simulink model "IRB140"  (R2019a)
settings: Solver=VariableStepAuto  StartTime=0.0  StopTime=10.0  RelTol=1e-3
InitFcn:
  | rpm_max=5000;
  | trq_stall=7;
  | T_i=1e-3;
  | eta=100;
  | rpm_eta=3000;
  | trq_eta=2.07;
  | J=0.672*1e-4;
  | rpm0=0;
  | gearRatio=10;
  | ts=0.0025;
undefined symbols (not defined in the file or in its folder): sigbuilder_block, X, Y, Z
libraries: sm_lib x61, fl_lib x42, nesl_utility x31, simulink x12, eeGeneralControl x12, ee_lib x6
(part 1 of 3)
settings Model: Creator=Richard urben  LastModifiedBy=Richard urben

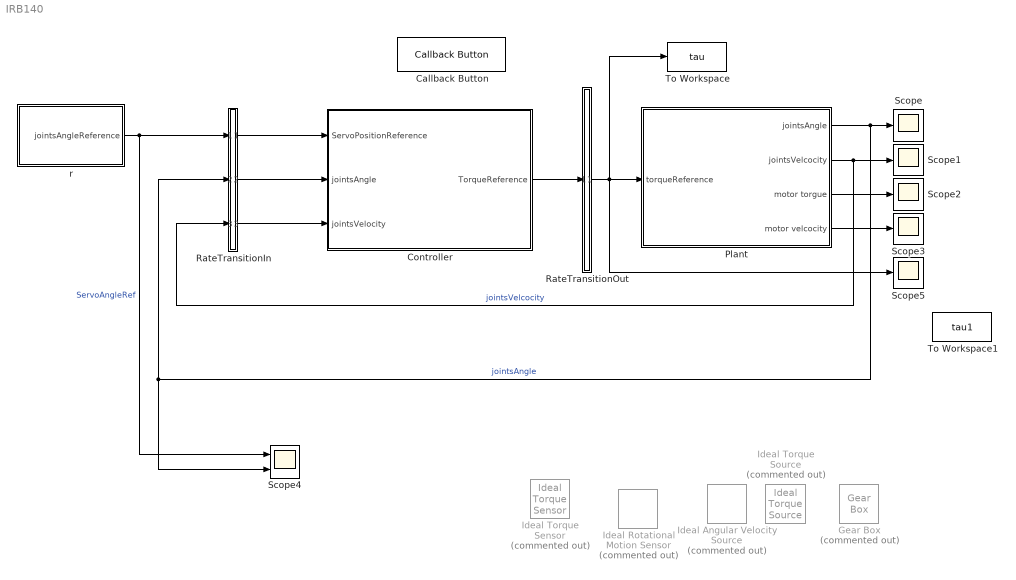
== system IRB140 ==
  Callback Button : CallbackButton  ButtonText=controler tuner
      settings: ClickFcn=|
      | h=0.005;
      | k=0.5;
      | controlParameters;
      | controlSystemTuner('ControlSystemTunerSession.mat');
  Controller : Subsystem
  Gear Box : fl_lib/Mechanical/Mechanisms/Gear Box  Commented=on  ratio=5  t_in_specify=off  t_in_priority=None  t_in=0 N*m  t_in_nominal_specify=off  t_in_nominal_unit=N*m  t_in_nominal_value=1  t_out_specify=off  t_out_priority=None  t_out=0 N*m  t_out_nominal_specify=off  t_out_nominal_unit=N*m  t_out_nominal_value=1
  Ideal Angular Velocity Source : fl_lib/Mechanical/Mechanical Sources/Ideal Angular Velocity Source  Commented=on
  Ideal Rotational Motion Sensor : fl_lib/Mechanical/Mechanical Sensors/Ideal Rotational Motion Sensor  Commented=on  offset=0 rad
  Ideal Torque Sensor : fl_lib/Mechanical/Mechanical Sensors/Ideal Torque Sensor  Commented=on
  Ideal Torque Source : fl_lib/Mechanical/Mechanical Sources/Ideal Torque Source  Commented=on
  Plant : Subsystem
  RateTransitionIn : Subsystem
  RateTransitionOut : Subsystem
  Scope{,1..3,5} (5 alike) : Scope
  Scope4 : Scope  NumInputPorts=2
  To Workspace : ToWorkspace  VariableName=tau  SaveFormat=Timeseries  SampleTime=2.5e-3
      settings: Decimation=6
  To Workspace1 : ToWorkspace  VariableName=tau1  SaveFormat=Timeseries  SampleTime=2.5e-3
      settings: Decimation=6
  r : Subsystem
      mask Display: disp('input')
  wires:
  Plant/2(jointsVelcocity) -> RateTransitionIn/3(joints_VelocityIn), Scope1/1  "jointsVelcocity"
  RateTransitionOut/1(tRef) -> Scope5/1, To Workspace/1, Plant/1(torqueReference)
  Controller/1(TorqueReference) -> RateTransitionOut/1(tRefIn)
  RateTransitionIn/1(ServoPositionRefOut) -> Controller/1(ServoPositionReference)
  RateTransitionIn/2(joints_AngleOut) -> Controller/2(jointsAngle)
  RateTransitionIn/3(joints_VelocityOut) -> Controller/3(jointsVelocity)
  Plant/1(jointsAngle) -> Scope4/2, RateTransitionIn/2(joints_AngleIn), Scope/1  "jointsAngle"
  r/1(jointsAngleReference) -> Scope4/1, RateTransitionIn/1(ServoPositionRefIn)  "ServoAngleRef"
  Plant/3(motor torgue) -> Scope2/1
  Plant/4(motor velcocity) -> Scope3/1

== system IRB140/Controller ==
  ServoPositionReference : Inport  Unit=deg  SampleTime=ts
  jointsAngle : Inport  Port=2  Unit=deg  SampleTime=ts
  jointsVelocity : Inport  Port=3  Unit=deg/s  SampleTime=ts
  Servomotor Position Controller : Subsystem
  Servomotor Speed Controller : Subsystem
  TorqueReference : Outport  Unit=N*m  SampleTime=ts
  wires:
  Servomotor Speed Controller/1(servo_Tref) -> TorqueReference/1  "Tref"
  jointsAngle/1 -> Servomotor Position Controller/2(joint_q)
  jointsVelocity/1 -> Servomotor Speed Controller/2(joint_qd)
  ServoPositionReference/1 -> Servomotor Position Controller/1(servon_qref)
  Servomotor Position Controller/1(servon_qdref) -> Servomotor Speed Controller/1(servon_qdref)  "servoqdref"

== system IRB140/Plant ==
  torqueReference : Inport  Unit=N*m
  DC Voltage Source : fl_lib/Electrical/Electrical Sources/DC Voltage Source  v0=12 V
  ERef Vcc : fl_lib/Electrical/Electrical Elements/Electrical Reference
      settings: SourceProductName=Foundation Library
  MRRef Motor : fl_lib/Mechanical/Rotational Elements/Mechanical Rotational Reference
      settings: SourceProductName=Foundation Library
  robot : Subsystem
  servo system : Subsystem
  jointsAngle : Outport  Unit=deg
  jointsVelcocity : Outport  Port=2  Unit=deg/s
  motor torgue : Outport  Port=3
  motor velcocity : Outport  Port=4
  wires:
  robot/2(w) -> jointsVelcocity/1  "jointsvelocity"
  robot/1(q) -> jointsAngle/1  "jointsangle"
  servo system/1(torque) -> motor torgue/1  "motor torque"
  servo system/2(motVel) -> motor velcocity/1  "motor velocity"
  torqueReference/1 -> servo system/1(tRef)
  connections:
  robot/LConn4 -- servo system/RConn4
  robot/LConn5 -- servo system/RConn5
  robot/LConn3 -- servo system/RConn3
  robot/LConn1 -- servo system/RConn1
  robot/LConn6 -- servo system/RConn6
  servo system/RConn7 -- MRRef Motor/LConn1 -- robot/LConn7
  robot/LConn2 -- servo system/RConn2
  ERef Vcc/LConn1 -- DC Voltage Source/RConn1 -- servo system/LConn2
  DC Voltage Source/LConn1 -- servo system/LConn1

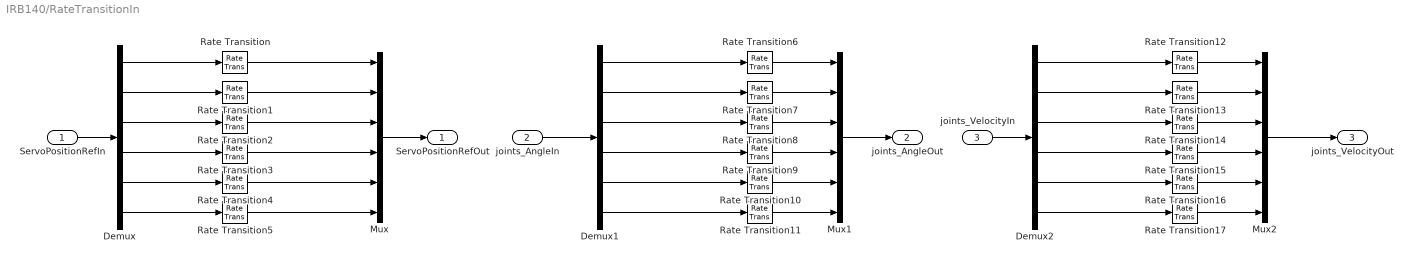
== system IRB140/RateTransitionIn ==
  ServoPositionRefIn : Inport  Unit=deg
  joints_AngleIn : Inport  Port=2  Unit=deg
  joints_VelocityIn : Inport  Port=3
  Demux : Demux  Outputs=6
  Demux1 : Demux  Outputs=6
  Demux2 : Demux  Outputs=6
  Mux : Mux  Inputs=6
  Mux1 : Mux  Inputs=6
  Mux2 : Mux  Inputs=6
  Rate Transition{,1..17} (18 alike) : RateTransition  OutPortSampleTime=ts
  ServoPositionRefOut : Outport
  joints_AngleOut : Outport  Port=2
  joints_VelocityOut : Outport  Port=3
  wires:
  Demux1/6 -> Rate Transition11/1
  Demux1/3 -> Rate Transition8/1
  joints_AngleIn/1 -> Demux1/1
  Demux1/1 -> Rate Transition6/1
  Demux1/5 -> Rate Transition10/1
  Demux/6 -> Rate Transition5/1
  Demux1/4 -> Rate Transition9/1
  Demux/2 -> Rate Transition1/1
  Demux1/2 -> Rate Transition7/1
  Demux/3 -> Rate Transition2/1
  Demux/4 -> Rate Transition3/1
  Demux/1 -> Rate Transition/1
  Demux/5 -> Rate Transition4/1
  Demux2/5 -> Rate Transition16/1
  Demux2/4 -> Rate Transition15/1
  Demux2/3 -> Rate Transition14/1
  Demux2/1 -> Rate Transition12/1
  Demux2/2 -> Rate Transition13/1
  Demux2/6 -> Rate Transition17/1
  Rate Transition/1 -> Mux/1
  Rate Transition1/1 -> Mux/2
  Rate Transition2/1 -> Mux/3
  Rate Transition3/1 -> Mux/4
  Rate Transition4/1 -> Mux/5
  Rate Transition5/1 -> Mux/6
  Mux/1 -> ServoPositionRefOut/1
  Rate Transition7/1 -> Mux1/2
  Rate Transition11/1 -> Mux1/6
  Mux1/1 -> joints_AngleOut/1
  Rate Transition9/1 -> Mux1/4
  Rate Transition6/1 -> Mux1/1
  Rate Transition8/1 -> Mux1/3
  Rate Transition10/1 -> Mux1/5
  Rate Transition12/1 -> Mux2/1
  Rate Transition13/1 -> Mux2/2
  Rate Transition14/1 -> Mux2/3
  Rate Transition15/1 -> Mux2/4
  Rate Transition16/1 -> Mux2/5
  Rate Transition17/1 -> Mux2/6
  Mux2/1 -> joints_VelocityOut/1
  ServoPositionRefIn/1 -> Demux/1
  joints_VelocityIn/1 -> Demux2/1

== system IRB140/RateTransitionOut ==
  tRefIn : Inport  Unit=N*m
  Demux : Demux  Outputs=6
  Mux : Mux  Inputs=6
  Zero-Order Hold{,1..5} (6 alike) : ZeroOrderHold  SampleTime=-1
  tRef : Outport  SampleTime=ts
  wires:
  Demux/3 -> Zero-Order Hold2/1
  tRefIn/1 -> Demux/1
  Demux/2 -> Zero-Order Hold1/1
  Demux/5 -> Zero-Order Hold4/1
  Demux/4 -> Zero-Order Hold3/1
  Demux/1 -> Zero-Order Hold/1
  Demux/6 -> Zero-Order Hold5/1
  Zero-Order Hold5/1 -> Mux/6
  Zero-Order Hold4/1 -> Mux/5
  Zero-Order Hold1/1 -> Mux/2
  Zero-Order Hold/1 -> Mux/1
  Zero-Order Hold2/1 -> Mux/3
  Zero-Order Hold3/1 -> Mux/4
  Mux/1 -> tRef/1

== system IRB140/r ==
  Mux : Mux  Commented=on  Inputs=6
  Mux1 : Mux  Inputs=6
  Subsystem : Subsystem
  Trajectories1 : Subsystem  Tag=STV Subsys  Commented=on  LoadFcn=sigbuilder_block('load');  StartFcn=sigbuilder_block('start');  StopFcn=sigbuilder_block('stop');  ClipboardFcn=sigbuilder_block('clipboard');  mask(Sigbuilder block){tuvar=[0:10]}
      mask help: Simulink:masks:SigbuilderBlock_MD
      mask init:
      | if ~strcmp(get_param(bdroot(gcbh),'SimulationStatus'),'stopped') tuvar = sigbuilder_block('maskInit'); end
      settings: CopyFcn=sigbuilder_block('copy');  DeleteFcn=sigbuilder_block('delete');  ModelCloseFcn=sigbuilder_block('modelClose');  PreSaveFcn=sigbuilder_block('preSave');  PauseFcn=sigbuilder_block('pause');  ContinueFcn=sigbuilder_block('continue');  NameChangeFcn=sigbuilder_block('namechange');  OpenFcn=sigbuilder_block('open',[6 -16.5 1248 598.5 ]);  CloseFcn=sigbuilder_block('close');
      mask Display: plot(0, 0, 100, 100,[2, 2, 32, 32, 2], [68, 8, 8, 68, 68],[32, 2], [38, 38], [32, 19, 2],[53, 60, 44], [32, 17, 17, 2],[16, 16, 31, 31]);txt = getActiveGroup(gcbh);text(2, 100, txt,'verticalAlignment', 'top');
  jointsAngleReference : Outport
  wires:
  Trajectories1/6(servopos6) -> Mux/6
  Trajectories1/2(servopos2) -> Mux/2
  Trajectories1/5(servopos5) -> Mux/5
  Trajectories1/1(servopos1) -> Mux/1
  Trajectories1/4(servopos4) -> Mux/4
  Trajectories1/3(servopos3) -> Mux/3
  Subsystem/5(Out5) -> Mux1/5
  Subsystem/1(Out1) -> Mux1/1
  Subsystem/3(Out3) -> Mux1/3
  Subsystem/2(Out2) -> Mux1/2
  Subsystem/6(Out6) -> Mux1/6
  Subsystem/4(Out4) -> Mux1/4
  Mux1/1 -> jointsAngleReference/1  "jointsAngleReferene"

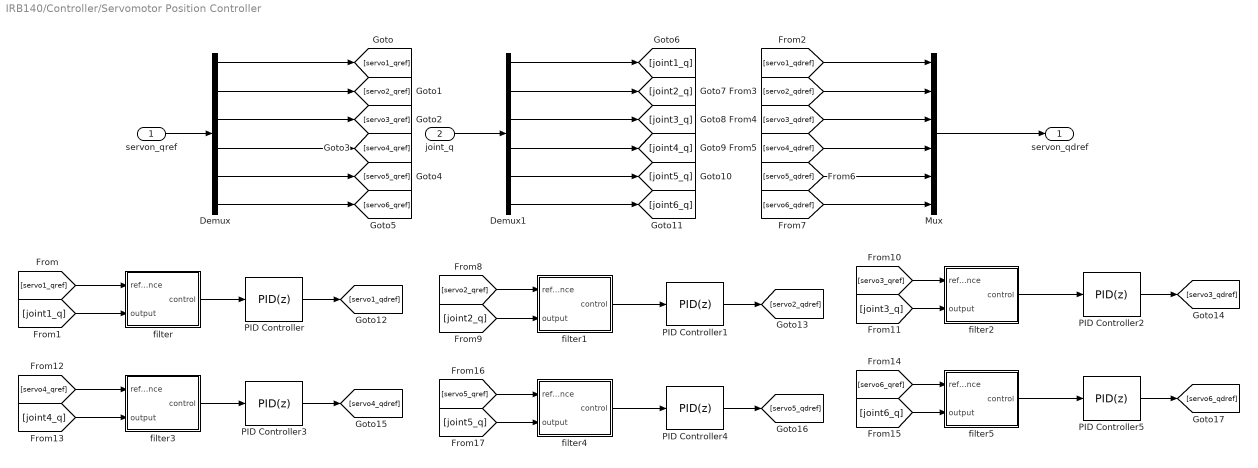
== system IRB140/Controller/Servomotor Position Controller ==
  servon_qref : Inport  Unit=deg
  joint_q : Inport  Port=2  Unit=deg
  Demux : Demux  Outputs=6
  Demux1 : Demux  Outputs=6
  Mux : Mux  Inputs=6
  PID Controller : simulink/Continuous/PID Controller  Controller=PID  Form=Parallel  TimeDomain=Discrete-time  SampleTime=ts  IntegratorMethod=Forward Euler  FilterMethod=Forward Euler  ControllerParametersSource=internal  P=9.61814981930867  I=0.000384969709550726  D=1.05281007023022  UseFilter=on  N=761.904761904762  TunerSelectOption=Transfer Function Based (PID Tuner App)  InitialConditionSource=internal  InitialConditionForIntegrator=0  InitialConditionForFilter=0  DifferentiatorICPrevScaledInput=0  ExternalReset=none  TrackingMode=off  Kt=1  LimitOutput=off  UpperSaturationLimit=inf  LowerSaturationLimit=-inf  LinearizeAsGain=on  AntiWindupMode=none  Kb=1  POutMin=[]  POutMax=[]  IOutMin=[]  IOutMax=[]  DOutMin=[]  DOutMax=[]  NOutMin=[]  NOutMax=[]  SumOutMin=[]  SumOutMax=[]  SaturationOutMin=[]  SaturationOutMax=[]  PParamMin=[]  PParamMax=[]  IParamMin=[]  IParamMax=[]  DParamMin=[]  DParamMax=[]  NParamMin=[]  NParamMax=[]  KbParamMin=[]  KbParamMax=[]  KtParamMin=[]  KtParamMax=[]  KbOutMin=[]  KbOutMax=[]  KtOutMin=[]  KtOutMax=[]  IntegratorOutMin=[]  IntegratorOutMax=[]  FilterOutMin=[]  FilterOutMax=[]  SumI1OutMin=[]  SumI1OutMax=[]  SumI2OutMin=[]  SumI2OutMax=[]  SumI3OutMin=[]  SumI3OutMax=[]  SumI4OutMin=[]  SumI4OutMax=[]  SumDOutMin=[]  SumDOutMax=[]  DifferentiatorOutMin=[]  DifferentiatorOutMax=[]  FilterDiffOutCoefMin=[]  FilterDiffOutCoefMax=[]  ReciprocalOutMin=[]  ReciprocalOutMax=[]  SumDenOutMin=[]  SumDenOutMax=[]  SumNumOutMin=[]  SumNumOutMax=[]  DivideOutMin=[]  DivideOutMax=[]  IntegratorContinuousStateAttributes=''  IntegratorStateMustResolveToSignalObject=off  IntegratorRTWStateStorageClass=Auto  FilterContinuousStateAttributes=''  FilterStateMustResolveToSignalObject=off  FilterRTWStateStorageClass=Auto  ParallelPVariant=InternalParameters  IdealPVariant=Disabled  IVariant=InternalParameters  DVariant=InternalParameters  IntegratorVariant=Discrete  SatVariant=Disabled  AWVariant=Passthrough  PCopyVariant=Disabled  TRVariant=Disabled  FdbkBlocksVariant=Forward  IdealPFdbkVariant=Disabled  SatFdbkVariant=Disabled  DerivativeFilterVariant=ForwardEulerFilter  NVariant=InternalParameters  NCopyVariant=Disabled  FilterICVariant=InternalICsFilter  IntegratorICVariant=InternalICs  ExternalResetVariant=Disabled  TRSumVariant=Passthrough  SumFdbkVariant=Disabled  SumVariant=Sum_PID
  PID Controller1 : simulink/Continuous/PID Controller  Controller=PID  Form=Parallel  TimeDomain=Discrete-time  SampleTime=ts  IntegratorMethod=Forward Euler  FilterMethod=Forward Euler  ControllerParametersSource=internal  P=7.83896752320748  I=0.000386528542327535  D=47.2359430142976  UseFilter=on  N=761.904761904762  TunerSelectOption=Transfer Function Based (PID Tuner App)  InitialConditionSource=internal  InitialConditionForIntegrator=0  InitialConditionForFilter=0  DifferentiatorICPrevScaledInput=0  ExternalReset=none  TrackingMode=off  Kt=1  LimitOutput=off  UpperSaturationLimit=inf  LowerSaturationLimit=-inf  LinearizeAsGain=on  AntiWindupMode=none  Kb=1  POutMin=[]  POutMax=[]  IOutMin=[]  IOutMax=[]  DOutMin=[]  DOutMax=[]  NOutMin=[]  NOutMax=[]  SumOutMin=[]  SumOutMax=[]  SaturationOutMin=[]  SaturationOutMax=[]  PParamMin=[]  PParamMax=[]  IParamMin=[]  IParamMax=[]  DParamMin=[]  DParamMax=[]  NParamMin=[]  NParamMax=[]  KbParamMin=[]  KbParamMax=[]  KtParamMin=[]  KtParamMax=[]  KbOutMin=[]  KbOutMax=[]  KtOutMin=[]  KtOutMax=[]  IntegratorOutMin=[]  IntegratorOutMax=[]  FilterOutMin=[]  FilterOutMax=[]  SumI1OutMin=[]  SumI1OutMax=[]  SumI2OutMin=[]  SumI2OutMax=[]  SumI3OutMin=[]  SumI3OutMax=[]  SumI4OutMin=[]  SumI4OutMax=[]  SumDOutMin=[]  SumDOutMax=[]  DifferentiatorOutMin=[]  DifferentiatorOutMax=[]  FilterDiffOutCoefMin=[]  FilterDiffOutCoefMax=[]  ReciprocalOutMin=[]  ReciprocalOutMax=[]  SumDenOutMin=[]  SumDenOutMax=[]  SumNumOutMin=[]  SumNumOutMax=[]  DivideOutMin=[]  DivideOutMax=[]  IntegratorContinuousStateAttributes=''  IntegratorStateMustResolveToSignalObject=off  IntegratorRTWStateStorageClass=Auto  FilterContinuousStateAttributes=''  FilterStateMustResolveToSignalObject=off  FilterRTWStateStorageClass=Auto  ParallelPVariant=InternalParameters  IdealPVariant=Disabled  IVariant=InternalParameters  DVariant=InternalParameters  IntegratorVariant=Discrete  SatVariant=Disabled  AWVariant=Passthrough  PCopyVariant=Disabled  TRVariant=Disabled  FdbkBlocksVariant=Forward  IdealPFdbkVariant=Disabled  SatFdbkVariant=Disabled  DerivativeFilterVariant=ForwardEulerFilter  NVariant=InternalParameters  NCopyVariant=Disabled  FilterICVariant=InternalICsFilter  IntegratorICVariant=InternalICs  ExternalResetVariant=Disabled  TRSumVariant=Passthrough  SumFdbkVariant=Disabled  SumVariant=Sum_PID
  PID Controller2 : simulink/Continuous/PID Controller  Controller=PID  Form=Parallel  TimeDomain=Discrete-time  SampleTime=ts  IntegratorMethod=Forward Euler  FilterMethod=Forward Euler  ControllerParametersSource=internal  P=10.5138297850177  I=0.000431195610304714  D=4.22368846435217  UseFilter=on  N=33.2552582353016  TunerSelectOption=Transfer Function Based (PID Tuner App)  InitialConditionSource=internal  InitialConditionForIntegrator=0  InitialConditionForFilter=0  DifferentiatorICPrevScaledInput=0  ExternalReset=none  TrackingMode=off  Kt=1  LimitOutput=off  UpperSaturationLimit=inf  LowerSaturationLimit=-inf  LinearizeAsGain=on  AntiWindupMode=none  Kb=1  POutMin=[]  POutMax=[]  IOutMin=[]  IOutMax=[]  DOutMin=[]  DOutMax=[]  NOutMin=[]  NOutMax=[]  SumOutMin=[]  SumOutMax=[]  SaturationOutMin=[]  SaturationOutMax=[]  PParamMin=[]  PParamMax=[]  IParamMin=[]  IParamMax=[]  DParamMin=[]  DParamMax=[]  NParamMin=[]  NParamMax=[]  KbParamMin=[]  KbParamMax=[]  KtParamMin=[]  KtParamMax=[]  KbOutMin=[]  KbOutMax=[]  KtOutMin=[]  KtOutMax=[]  IntegratorOutMin=[]  IntegratorOutMax=[]  FilterOutMin=[]  FilterOutMax=[]  SumI1OutMin=[]  SumI1OutMax=[]  SumI2OutMin=[]  SumI2OutMax=[]  SumI3OutMin=[]  SumI3OutMax=[]  SumI4OutMin=[]  SumI4OutMax=[]  SumDOutMin=[]  SumDOutMax=[]  DifferentiatorOutMin=[]  DifferentiatorOutMax=[]  FilterDiffOutCoefMin=[]  FilterDiffOutCoefMax=[]  ReciprocalOutMin=[]  ReciprocalOutMax=[]  SumDenOutMin=[]  SumDenOutMax=[]  SumNumOutMin=[]  SumNumOutMax=[]  DivideOutMin=[]  DivideOutMax=[]  IntegratorContinuousStateAttributes=''  IntegratorStateMustResolveToSignalObject=off  IntegratorRTWStateStorageClass=Auto  FilterContinuousStateAttributes=''  FilterStateMustResolveToSignalObject=off  FilterRTWStateStorageClass=Auto  ParallelPVariant=InternalParameters  IdealPVariant=Disabled  IVariant=InternalParameters  DVariant=InternalParameters  IntegratorVariant=Discrete  SatVariant=Disabled  AWVariant=Passthrough  PCopyVariant=Disabled  TRVariant=Disabled  FdbkBlocksVariant=Forward  IdealPFdbkVariant=Disabled  SatFdbkVariant=Disabled  DerivativeFilterVariant=ForwardEulerFilter  NVariant=InternalParameters  NCopyVariant=Disabled  FilterICVariant=InternalICsFilter  IntegratorICVariant=InternalICs  ExternalResetVariant=Disabled  TRSumVariant=Passthrough  SumFdbkVariant=Disabled  SumVariant=Sum_PID
  PID Controller3 : simulink/Continuous/PID Controller  Controller=PID  Form=Parallel  TimeDomain=Discrete-time  SampleTime=ts  IntegratorMethod=Forward Euler  FilterMethod=Forward Euler  ControllerParametersSource=internal  P=11.567292222451  I=0.0350806139958513  D=64.3949997246257  UseFilter=on  N=761.904761904762  TunerSelectOption=Transfer Function Based (PID Tuner App)  InitialConditionSource=internal  InitialConditionForIntegrator=0  InitialConditionForFilter=0  DifferentiatorICPrevScaledInput=0  ExternalReset=none  TrackingMode=off  Kt=1  LimitOutput=off  UpperSaturationLimit=inf  LowerSaturationLimit=-inf  LinearizeAsGain=on  AntiWindupMode=none  Kb=1  POutMin=[]  POutMax=[]  IOutMin=[]  IOutMax=[]  DOutMin=[]  DOutMax=[]  NOutMin=[]  NOutMax=[]  SumOutMin=[]  SumOutMax=[]  SaturationOutMin=[]  SaturationOutMax=[]  PParamMin=[]  PParamMax=[]  IParamMin=[]  IParamMax=[]  DParamMin=[]  DParamMax=[]  NParamMin=[]  NParamMax=[]  KbParamMin=[]  KbParamMax=[]  KtParamMin=[]  KtParamMax=[]  KbOutMin=[]  KbOutMax=[]  KtOutMin=[]  KtOutMax=[]  IntegratorOutMin=[]  IntegratorOutMax=[]  FilterOutMin=[]  FilterOutMax=[]  SumI1OutMin=[]  SumI1OutMax=[]  SumI2OutMin=[]  SumI2OutMax=[]  SumI3OutMin=[]  SumI3OutMax=[]  SumI4OutMin=[]  SumI4OutMax=[]  SumDOutMin=[]  SumDOutMax=[]  DifferentiatorOutMin=[]  DifferentiatorOutMax=[]  FilterDiffOutCoefMin=[]  FilterDiffOutCoefMax=[]  ReciprocalOutMin=[]  ReciprocalOutMax=[]  SumDenOutMin=[]  SumDenOutMax=[]  SumNumOutMin=[]  SumNumOutMax=[]  DivideOutMin=[]  DivideOutMax=[]  IntegratorContinuousStateAttributes=''  IntegratorStateMustResolveToSignalObject=off  IntegratorRTWStateStorageClass=Auto  FilterContinuousStateAttributes=''  FilterStateMustResolveToSignalObject=off  FilterRTWStateStorageClass=Auto  ParallelPVariant=InternalParameters  IdealPVariant=Disabled  IVariant=InternalParameters  DVariant=InternalParameters  IntegratorVariant=Discrete  SatVariant=Disabled  AWVariant=Passthrough  PCopyVariant=Disabled  TRVariant=Disabled  FdbkBlocksVariant=Forward  IdealPFdbkVariant=Disabled  SatFdbkVariant=Disabled  DerivativeFilterVariant=ForwardEulerFilter  NVariant=InternalParameters  NCopyVariant=Disabled  FilterICVariant=InternalICsFilter  IntegratorICVariant=InternalICs  ExternalResetVariant=Disabled  TRSumVariant=Passthrough  SumFdbkVariant=Disabled  SumVariant=Sum_PID
  PID Controller4 : simulink/Continuous/PID Controller  Controller=PID  Form=Parallel  TimeDomain=Discrete-time  SampleTime=ts  IntegratorMethod=Forward Euler  FilterMethod=Forward Euler  ControllerParametersSource=internal  P=10.5558393494834  I=0.000423023219587535  D=1077.75365309881  UseFilter=on  N=0.000227846828002972  TunerSelectOption=Transfer Function Based (PID Tuner App)  InitialConditionSource=internal  InitialConditionForIntegrator=0  InitialConditionForFilter=0  DifferentiatorICPrevScaledInput=0  ExternalReset=none  TrackingMode=off  Kt=1  LimitOutput=off  UpperSaturationLimit=inf  LowerSaturationLimit=-inf  LinearizeAsGain=on  AntiWindupMode=none  Kb=1  POutMin=[]  POutMax=[]  IOutMin=[]  IOutMax=[]  DOutMin=[]  DOutMax=[]  NOutMin=[]  NOutMax=[]  SumOutMin=[]  SumOutMax=[]  SaturationOutMin=[]  SaturationOutMax=[]  PParamMin=[]  PParamMax=[]  IParamMin=[]  IParamMax=[]  DParamMin=[]  DParamMax=[]  NParamMin=[]  NParamMax=[]  KbParamMin=[]  KbParamMax=[]  KtParamMin=[]  KtParamMax=[]  KbOutMin=[]  KbOutMax=[]  KtOutMin=[]  KtOutMax=[]  IntegratorOutMin=[]  IntegratorOutMax=[]  FilterOutMin=[]  FilterOutMax=[]  SumI1OutMin=[]  SumI1OutMax=[]  SumI2OutMin=[]  SumI2OutMax=[]  SumI3OutMin=[]  SumI3OutMax=[]  SumI4OutMin=[]  SumI4OutMax=[]  SumDOutMin=[]  SumDOutMax=[]  DifferentiatorOutMin=[]  DifferentiatorOutMax=[]  FilterDiffOutCoefMin=[]  FilterDiffOutCoefMax=[]  ReciprocalOutMin=[]  ReciprocalOutMax=[]  SumDenOutMin=[]  SumDenOutMax=[]  SumNumOutMin=[]  SumNumOutMax=[]  DivideOutMin=[]  DivideOutMax=[]  IntegratorContinuousStateAttributes=''  IntegratorStateMustResolveToSignalObject=off  IntegratorRTWStateStorageClass=Auto  FilterContinuousStateAttributes=''  FilterStateMustResolveToSignalObject=off  FilterRTWStateStorageClass=Auto  ParallelPVariant=InternalParameters  IdealPVariant=Disabled  IVariant=InternalParameters  DVariant=InternalParameters  IntegratorVariant=Discrete  SatVariant=Disabled  AWVariant=Passthrough  PCopyVariant=Disabled  TRVariant=Disabled  FdbkBlocksVariant=Forward  IdealPFdbkVariant=Disabled  SatFdbkVariant=Disabled  DerivativeFilterVariant=ForwardEulerFilter  NVariant=InternalParameters  NCopyVariant=Disabled  FilterICVariant=InternalICsFilter  IntegratorICVariant=InternalICs  ExternalResetVariant=Disabled  TRSumVariant=Passthrough  SumFdbkVariant=Disabled  SumVariant=Sum_PID
  PID Controller5 : simulink/Continuous/PID Controller  Controller=PID  Form=Parallel  TimeDomain=Discrete-time  SampleTime=ts  IntegratorMethod=Forward Euler  FilterMethod=Forward Euler  ControllerParametersSource=internal  P=10.7489084573327  I=0.000565481072663244  D=0.219267845296139  UseFilter=on  N=148.133193583419  TunerSelectOption=Transfer Function Based (PID Tuner App)  InitialConditionSource=internal  InitialConditionForIntegrator=0  InitialConditionForFilter=0  DifferentiatorICPrevScaledInput=0  ExternalReset=none  TrackingMode=off  Kt=1  LimitOutput=off  UpperSaturationLimit=inf  LowerSaturationLimit=-inf  LinearizeAsGain=on  AntiWindupMode=none  Kb=1  POutMin=[]  POutMax=[]  IOutMin=[]  IOutMax=[]  DOutMin=[]  DOutMax=[]  NOutMin=[]  NOutMax=[]  SumOutMin=[]  SumOutMax=[]  SaturationOutMin=[]  SaturationOutMax=[]  PParamMin=[]  PParamMax=[]  IParamMin=[]  IParamMax=[]  DParamMin=[]  DParamMax=[]  NParamMin=[]  NParamMax=[]  KbParamMin=[]  KbParamMax=[]  KtParamMin=[]  KtParamMax=[]  KbOutMin=[]  KbOutMax=[]  KtOutMin=[]  KtOutMax=[]  IntegratorOutMin=[]  IntegratorOutMax=[]  FilterOutMin=[]  FilterOutMax=[]  SumI1OutMin=[]  SumI1OutMax=[]  SumI2OutMin=[]  SumI2OutMax=[]  SumI3OutMin=[]  SumI3OutMax=[]  SumI4OutMin=[]  SumI4OutMax=[]  SumDOutMin=[]  SumDOutMax=[]  DifferentiatorOutMin=[]  DifferentiatorOutMax=[]  FilterDiffOutCoefMin=[]  FilterDiffOutCoefMax=[]  ReciprocalOutMin=[]  ReciprocalOutMax=[]  SumDenOutMin=[]  SumDenOutMax=[]  SumNumOutMin=[]  SumNumOutMax=[]  DivideOutMin=[]  DivideOutMax=[]  IntegratorContinuousStateAttributes=''  IntegratorStateMustResolveToSignalObject=off  IntegratorRTWStateStorageClass=Auto  FilterContinuousStateAttributes=''  FilterStateMustResolveToSignalObject=off  FilterRTWStateStorageClass=Auto  ParallelPVariant=InternalParameters  IdealPVariant=Disabled  IVariant=InternalParameters  DVariant=InternalParameters  IntegratorVariant=Discrete  SatVariant=Disabled  AWVariant=Passthrough  PCopyVariant=Disabled  TRVariant=Disabled  FdbkBlocksVariant=Forward  IdealPFdbkVariant=Disabled  SatFdbkVariant=Disabled  DerivativeFilterVariant=ForwardEulerFilter  NVariant=InternalParameters  NCopyVariant=Disabled  FilterICVariant=InternalICsFilter  IntegratorICVariant=InternalICs  ExternalResetVariant=Disabled  TRSumVariant=Passthrough  SumFdbkVariant=Disabled  SumVariant=Sum_PID
  filter : Subsystem
  filter1 : Subsystem
  filter2 : Subsystem
  filter3 : Subsystem
  filter4 : Subsystem
  filter5 : Subsystem
  servon_qdref : Outport  Unit=deg/s
  wires:
  PID Controller/1 -> [servo1_qdref]
  [joint5_q] -> filter4/2(output)
  Demux/3 -> [servo3_qref]
  Demux/6 -> [servo6_qref]
  Demux/5 -> [servo5_qref]
  Demux/4 -> [servo4_qref]
  Demux1/3 -> [joint3_q]
  Demux/2 -> [servo2_qref]
  filter4/1(control) -> PID Controller4/1
  [servo2_qdref] -> Mux/2
  Demux1/2 -> [joint2_q]
  joint_q/1 -> Demux1/1
  Demux/1 -> [servo1_qref]
  [servo1_qref] -> filter/1(reference)
  Demux1/6 -> [joint6_q]
  [servo2_qref] -> filter1/1(reference)
  filter3/1(control) -> PID Controller3/1
  [joint6_q] -> filter5/2(output)
  Demux1/4 -> [joint4_q]
  servon_qref/1 -> Demux/1
  Demux1/5 -> [joint5_q]
  filter/1(control) -> PID Controller/1
  Demux1/1 -> [joint1_q]
  PID Controller5/1 -> [servo6_qdref]
  [servo1_qdref] -> Mux/1
  PID Controller2/1 -> [servo3_qdref]
  [servo5_qdref] -> Mux/5
  [servo4_qdref] -> Mux/4
  [servo6_qdref] -> Mux/6
  [servo3_qdref] -> Mux/3
  [joint1_q] -> filter/2(output)
  [joint2_q] -> filter1/2(output)
  Mux/1 -> servon_qdref/1
  PID Controller1/1 -> [servo2_qdref]
  filter1/1(control) -> PID Controller1/1
  filter2/1(control) -> PID Controller2/1
  PID Controller3/1 -> [servo4_qdref]
  PID Controller4/1 -> [servo5_qdref]
  [servo6_qref] -> filter5/1(reference)
  [servo5_qref] -> filter4/1(reference)
  [joint3_q] -> filter2/2(output)
  [servo3_qref] -> filter2/1(reference)
  [servo4_qref] -> filter3/1(reference)
  [joint4_q] -> filter3/2(output)
  filter5/1(control) -> PID Controller5/1

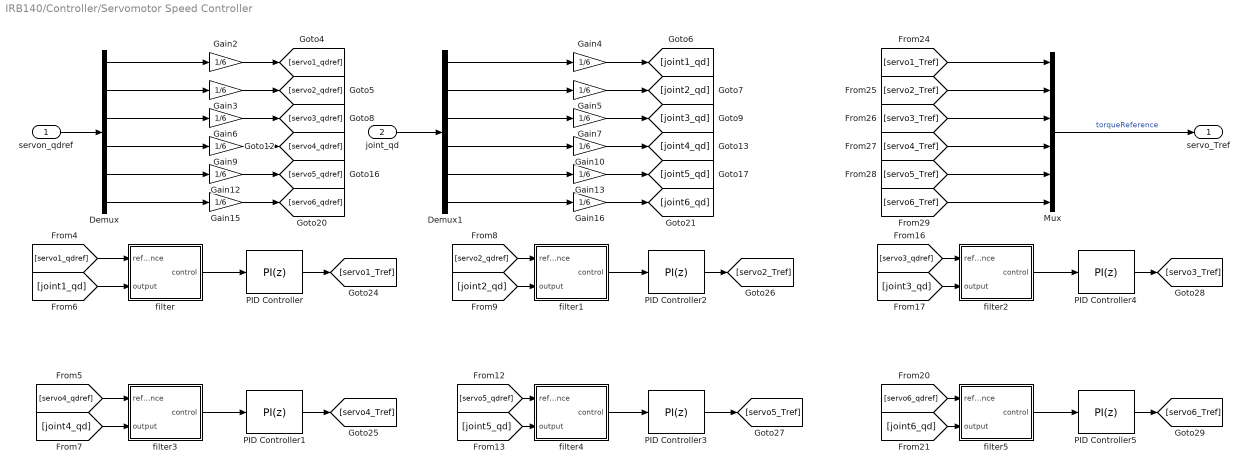
== system IRB140/Controller/Servomotor Speed Controller ==
  servon_qdref : Inport
  joint_qd : Inport  Port=2
  Demux : Demux  Outputs=6
  Demux1 : Demux  Outputs=6
  Gain{2..7,9..10,12..13,15..16} (12 alike) : Gain  Gain=1/6
  Mux : Mux  Inputs=6
  PID Controller : simulink/Continuous/PID Controller  Controller=PI  Form=Parallel  TimeDomain=Discrete-time  SampleTime=ts  IntegratorMethod=Forward Euler  FilterMethod=Forward Euler  ControllerParametersSource=internal  P=0.230491872560816  I=2.80022996495276e-05  D=0  UseFilter=on  N=0  TunerSelectOption=Transfer Function Based (PID Tuner App)  InitialConditionSource=internal  InitialConditionForIntegrator=0  InitialConditionForFilter=0  DifferentiatorICPrevScaledInput=0  ExternalReset=none  TrackingMode=off  Kt=1  LimitOutput=off  UpperSaturationLimit=inf  LowerSaturationLimit=-inf  LinearizeAsGain=on  AntiWindupMode=none  Kb=1  POutMin=[]  POutMax=[]  IOutMin=[]  IOutMax=[]  DOutMin=[]  DOutMax=[]  NOutMin=[]  NOutMax=[]  SumOutMin=[]  SumOutMax=[]  SaturationOutMin=[]  SaturationOutMax=[]  PParamMin=[]  PParamMax=[]  IParamMin=[]  IParamMax=[]  DParamMin=[]  DParamMax=[]  NParamMin=[]  NParamMax=[]  KbParamMin=[]  KbParamMax=[]  KtParamMin=[]  KtParamMax=[]  KbOutMin=[]  KbOutMax=[]  KtOutMin=[]  KtOutMax=[]  IntegratorOutMin=[]  IntegratorOutMax=[]  FilterOutMin=[]  FilterOutMax=[]  SumI1OutMin=[]  SumI1OutMax=[]  SumI2OutMin=[]  SumI2OutMax=[]  SumI3OutMin=[]  SumI3OutMax=[]  SumI4OutMin=[]  SumI4OutMax=[]  SumDOutMin=[]  SumDOutMax=[]  DifferentiatorOutMin=[]  DifferentiatorOutMax=[]  FilterDiffOutCoefMin=[]  FilterDiffOutCoefMax=[]  ReciprocalOutMin=[]  ReciprocalOutMax=[]  SumDenOutMin=[]  SumDenOutMax=[]  SumNumOutMin=[]  SumNumOutMax=[]  DivideOutMin=[]  DivideOutMax=[]  IntegratorContinuousStateAttributes=''  IntegratorStateMustResolveToSignalObject=off  IntegratorRTWStateStorageClass=Auto  FilterContinuousStateAttributes=''  FilterStateMustResolveToSignalObject=off  FilterRTWStateStorageClass=Auto  ParallelPVariant=InternalParameters  IdealPVariant=Disabled  IVariant=InternalParameters  DVariant=Disabled  IntegratorVariant=Discrete  SatVariant=Disabled  AWVariant=Passthrough  PCopyVariant=Disabled  TRVariant=Disabled  FdbkBlocksVariant=Forward  IdealPFdbkVariant=Disabled  SatFdbkVariant=Disabled  DerivativeFilterVariant=Disabled  NVariant=Disabled  NCopyVariant=Disabled_SignalSpec  FilterICVariant=Disabled  IntegratorICVariant=InternalICs  ExternalResetVariant=Disabled  TRSumVariant=Passthrough  SumFdbkVariant=Disabled  SumVariant=Sum_PI
  PID Controller1 : simulink/Continuous/PID Controller  Controller=PI  Form=Parallel  TimeDomain=Discrete-time  SampleTime=ts  IntegratorMethod=Forward Euler  FilterMethod=Forward Euler  ControllerParametersSource=internal  P=0.00294076623248856  I=2.32589389201061e-06  D=0  UseFilter=on  N=0  TunerSelectOption=Transfer Function Based (PID Tuner App)  InitialConditionSource=internal  InitialConditionForIntegrator=0  InitialConditionForFilter=0  DifferentiatorICPrevScaledInput=0  ExternalReset=none  TrackingMode=off  Kt=1  LimitOutput=off  UpperSaturationLimit=inf  LowerSaturationLimit=-inf  LinearizeAsGain=on  AntiWindupMode=none  Kb=1  POutMin=[]  POutMax=[]  IOutMin=[]  IOutMax=[]  DOutMin=[]  DOutMax=[]  NOutMin=[]  NOutMax=[]  SumOutMin=[]  SumOutMax=[]  SaturationOutMin=[]  SaturationOutMax=[]  PParamMin=[]  PParamMax=[]  IParamMin=[]  IParamMax=[]  DParamMin=[]  DParamMax=[]  NParamMin=[]  NParamMax=[]  KbParamMin=[]  KbParamMax=[]  KtParamMin=[]  KtParamMax=[]  KbOutMin=[]  KbOutMax=[]  KtOutMin=[]  KtOutMax=[]  IntegratorOutMin=[]  IntegratorOutMax=[]  FilterOutMin=[]  FilterOutMax=[]  SumI1OutMin=[]  SumI1OutMax=[]  SumI2OutMin=[]  SumI2OutMax=[]  SumI3OutMin=[]  SumI3OutMax=[]  SumI4OutMin=[]  SumI4OutMax=[]  SumDOutMin=[]  SumDOutMax=[]  DifferentiatorOutMin=[]  DifferentiatorOutMax=[]  FilterDiffOutCoefMin=[]  FilterDiffOutCoefMax=[]  ReciprocalOutMin=[]  ReciprocalOutMax=[]  SumDenOutMin=[]  SumDenOutMax=[]  SumNumOutMin=[]  SumNumOutMax=[]  DivideOutMin=[]  DivideOutMax=[]  IntegratorContinuousStateAttributes=''  IntegratorStateMustResolveToSignalObject=off  IntegratorRTWStateStorageClass=Auto  FilterContinuousStateAttributes=''  FilterStateMustResolveToSignalObject=off  FilterRTWStateStorageClass=Auto  ParallelPVariant=InternalParameters  IdealPVariant=Disabled  IVariant=InternalParameters  DVariant=Disabled  IntegratorVariant=Discrete  SatVariant=Disabled  AWVariant=Passthrough  PCopyVariant=Disabled  TRVariant=Disabled  FdbkBlocksVariant=Forward  IdealPFdbkVariant=Disabled  SatFdbkVariant=Disabled  DerivativeFilterVariant=Disabled  NVariant=Disabled  NCopyVariant=Disabled_SignalSpec  FilterICVariant=Disabled  IntegratorICVariant=InternalICs  ExternalResetVariant=Disabled  TRSumVariant=Passthrough  SumFdbkVariant=Disabled  SumVariant=Sum_PI
  PID Controller2 : simulink/Continuous/PID Controller  Controller=PI  Form=Parallel  TimeDomain=Discrete-time  SampleTime=ts  IntegratorMethod=Forward Euler  FilterMethod=Forward Euler  ControllerParametersSource=internal  P=0.0242233142132692  I=9.69554235497484e-07  D=0  UseFilter=on  N=0  TunerSelectOption=Transfer Function Based (PID Tuner App)  InitialConditionSource=internal  InitialConditionForIntegrator=0  InitialConditionForFilter=0  DifferentiatorICPrevScaledInput=0  ExternalReset=none  TrackingMode=off  Kt=1  LimitOutput=off  UpperSaturationLimit=inf  LowerSaturationLimit=-inf  LinearizeAsGain=on  AntiWindupMode=none  Kb=1  POutMin=[]  POutMax=[]  IOutMin=[]  IOutMax=[]  DOutMin=[]  DOutMax=[]  NOutMin=[]  NOutMax=[]  SumOutMin=[]  SumOutMax=[]  SaturationOutMin=[]  SaturationOutMax=[]  PParamMin=[]  PParamMax=[]  IParamMin=[]  IParamMax=[]  DParamMin=[]  DParamMax=[]  NParamMin=[]  NParamMax=[]  KbParamMin=[]  KbParamMax=[]  KtParamMin=[]  KtParamMax=[]  KbOutMin=[]  KbOutMax=[]  KtOutMin=[]  KtOutMax=[]  IntegratorOutMin=[]  IntegratorOutMax=[]  FilterOutMin=[]  FilterOutMax=[]  SumI1OutMin=[]  SumI1OutMax=[]  SumI2OutMin=[]  SumI2OutMax=[]  SumI3OutMin=[]  SumI3OutMax=[]  SumI4OutMin=[]  SumI4OutMax=[]  SumDOutMin=[]  SumDOutMax=[]  DifferentiatorOutMin=[]  DifferentiatorOutMax=[]  FilterDiffOutCoefMin=[]  FilterDiffOutCoefMax=[]  ReciprocalOutMin=[]  ReciprocalOutMax=[]  SumDenOutMin=[]  SumDenOutMax=[]  SumNumOutMin=[]  SumNumOutMax=[]  DivideOutMin=[]  DivideOutMax=[]  IntegratorContinuousStateAttributes=''  IntegratorStateMustResolveToSignalObject=off  IntegratorRTWStateStorageClass=Auto  FilterContinuousStateAttributes=''  FilterStateMustResolveToSignalObject=off  FilterRTWStateStorageClass=Auto  ParallelPVariant=InternalParameters  IdealPVariant=Disabled  IVariant=InternalParameters  DVariant=Disabled  IntegratorVariant=Discrete  SatVariant=Disabled  AWVariant=Passthrough  PCopyVariant=Disabled  TRVariant=Disabled  FdbkBlocksVariant=Forward  IdealPFdbkVariant=Disabled  SatFdbkVariant=Disabled  DerivativeFilterVariant=Disabled  NVariant=Disabled  NCopyVariant=Disabled_SignalSpec  FilterICVariant=Disabled  IntegratorICVariant=InternalICs  ExternalResetVariant=Disabled  TRSumVariant=Passthrough  SumFdbkVariant=Disabled  SumVariant=Sum_PI
  PID Controller3 : simulink/Continuous/PID Controller  Controller=PI  Form=Parallel  TimeDomain=Discrete-time  SampleTime=ts  IntegratorMethod=Forward Euler  FilterMethod=Forward Euler  ControllerParametersSource=internal  P=0.336205569865457  I=2.30915072791741  D=0  UseFilter=on  N=0  TunerSelectOption=Transfer Function Based (PID Tuner App)  InitialConditionSource=internal  InitialConditionForIntegrator=0  InitialConditionForFilter=0  DifferentiatorICPrevScaledInput=0  ExternalReset=none  TrackingMode=off  Kt=1  LimitOutput=off  UpperSaturationLimit=inf  LowerSaturationLimit=-inf  LinearizeAsGain=on  AntiWindupMode=none  Kb=1  POutMin=[]  POutMax=[]  IOutMin=[]  IOutMax=[]  DOutMin=[]  DOutMax=[]  NOutMin=[]  NOutMax=[]  SumOutMin=[]  SumOutMax=[]  SaturationOutMin=[]  SaturationOutMax=[]  PParamMin=[]  PParamMax=[]  IParamMin=[]  IParamMax=[]  DParamMin=[]  DParamMax=[]  NParamMin=[]  NParamMax=[]  KbParamMin=[]  KbParamMax=[]  KtParamMin=[]  KtParamMax=[]  KbOutMin=[]  KbOutMax=[]  KtOutMin=[]  KtOutMax=[]  IntegratorOutMin=[]  IntegratorOutMax=[]  FilterOutMin=[]  FilterOutMax=[]  SumI1OutMin=[]  SumI1OutMax=[]  SumI2OutMin=[]  SumI2OutMax=[]  SumI3OutMin=[]  SumI3OutMax=[]  SumI4OutMin=[]  SumI4OutMax=[]  SumDOutMin=[]  SumDOutMax=[]  DifferentiatorOutMin=[]  DifferentiatorOutMax=[]  FilterDiffOutCoefMin=[]  FilterDiffOutCoefMax=[]  ReciprocalOutMin=[]  ReciprocalOutMax=[]  SumDenOutMin=[]  SumDenOutMax=[]  SumNumOutMin=[]  SumNumOutMax=[]  DivideOutMin=[]  DivideOutMax=[]  IntegratorContinuousStateAttributes=''  IntegratorStateMustResolveToSignalObject=off  IntegratorRTWStateStorageClass=Auto  FilterContinuousStateAttributes=''  FilterStateMustResolveToSignalObject=off  FilterRTWStateStorageClass=Auto  ParallelPVariant=InternalParameters  IdealPVariant=Disabled  IVariant=InternalParameters  DVariant=Disabled  IntegratorVariant=Discrete  SatVariant=Disabled  AWVariant=Passthrough  PCopyVariant=Disabled  TRVariant=Disabled  FdbkBlocksVariant=Forward  IdealPFdbkVariant=Disabled  SatFdbkVariant=Disabled  DerivativeFilterVariant=Disabled  NVariant=Disabled  NCopyVariant=Disabled_SignalSpec  FilterICVariant=Disabled  IntegratorICVariant=InternalICs  ExternalResetVariant=Disabled  TRSumVariant=Passthrough  SumFdbkVariant=Disabled  SumVariant=Sum_PI
  PID Controller4 : simulink/Continuous/PID Controller  Controller=PI  Form=Parallel  TimeDomain=Discrete-time  SampleTime=ts  IntegratorMethod=Forward Euler  FilterMethod=Forward Euler  ControllerParametersSource=internal  P=0.148308871305365  I=5.93615803975065e-06  D=0  UseFilter=on  N=0  TunerSelectOption=Transfer Function Based (PID Tuner App)  InitialConditionSource=internal  InitialConditionForIntegrator=0  InitialConditionForFilter=0  DifferentiatorICPrevScaledInput=0  ExternalReset=none  TrackingMode=off  Kt=1  LimitOutput=off  UpperSaturationLimit=0.001  LowerSaturationLimit=-0.001  LinearizeAsGain=on  AntiWindupMode=none  Kb=1  POutMin=[]  POutMax=[]  IOutMin=[]  IOutMax=[]  DOutMin=[]  DOutMax=[]  NOutMin=[]  NOutMax=[]  SumOutMin=[]  SumOutMax=[]  SaturationOutMin=[]  SaturationOutMax=[]  PParamMin=[]  PParamMax=[]  IParamMin=[]  IParamMax=[]  DParamMin=[]  DParamMax=[]  NParamMin=[]  NParamMax=[]  KbParamMin=[]  KbParamMax=[]  KtParamMin=[]  KtParamMax=[]  KbOutMin=[]  KbOutMax=[]  KtOutMin=[]  KtOutMax=[]  IntegratorOutMin=[]  IntegratorOutMax=[]  FilterOutMin=[]  FilterOutMax=[]  SumI1OutMin=[]  SumI1OutMax=[]  SumI2OutMin=[]  SumI2OutMax=[]  SumI3OutMin=[]  SumI3OutMax=[]  SumI4OutMin=[]  SumI4OutMax=[]  SumDOutMin=[]  SumDOutMax=[]  DifferentiatorOutMin=[]  DifferentiatorOutMax=[]  FilterDiffOutCoefMin=[]  FilterDiffOutCoefMax=[]  ReciprocalOutMin=[]  ReciprocalOutMax=[]  SumDenOutMin=[]  SumDenOutMax=[]  SumNumOutMin=[]  SumNumOutMax=[]  DivideOutMin=[]  DivideOutMax=[]  IntegratorContinuousStateAttributes=''  IntegratorStateMustResolveToSignalObject=off  IntegratorRTWStateStorageClass=Auto  FilterContinuousStateAttributes=''  FilterStateMustResolveToSignalObject=off  FilterRTWStateStorageClass=Auto  ParallelPVariant=InternalParameters  IdealPVariant=Disabled  IVariant=InternalParameters  DVariant=Disabled  IntegratorVariant=Discrete  SatVariant=Disabled  AWVariant=Passthrough  PCopyVariant=Disabled  TRVariant=Disabled  FdbkBlocksVariant=Forward  IdealPFdbkVariant=Disabled  SatFdbkVariant=Disabled  DerivativeFilterVariant=Disabled  NVariant=Disabled  NCopyVariant=Disabled_SignalSpec  FilterICVariant=Disabled  IntegratorICVariant=InternalICs  ExternalResetVariant=Disabled  TRSumVariant=Passthrough  SumFdbkVariant=Disabled  SumVariant=Sum_PI
  PID Controller5 : simulink/Continuous/PID Controller  Controller=PI  Form=Parallel  TimeDomain=Discrete-time  SampleTime=ts  IntegratorMethod=Forward Euler  FilterMethod=Forward Euler  ControllerParametersSource=internal  P=0.0978663458019394  I=6.7878177642195e-06  D=0  UseFilter=on  N=0  TunerSelectOption=Transfer Function Based (PID Tuner App)  InitialConditionSource=internal  InitialConditionForIntegrator=0  InitialConditionForFilter=0  DifferentiatorICPrevScaledInput=0  ExternalReset=none  TrackingMode=off  Kt=1  LimitOutput=off  UpperSaturationLimit=0.001  LowerSaturationLimit=-0.001  LinearizeAsGain=on  AntiWindupMode=none  Kb=1  POutMin=[]  POutMax=[]  IOutMin=[]  IOutMax=[]  DOutMin=[]  DOutMax=[]  NOutMin=[]  NOutMax=[]  SumOutMin=[]  SumOutMax=[]  SaturationOutMin=[]  SaturationOutMax=[]  PParamMin=[]  PParamMax=[]  IParamMin=[]  IParamMax=[]  DParamMin=[]  DParamMax=[]  NParamMin=[]  NParamMax=[]  KbParamMin=[]  KbParamMax=[]  KtParamMin=[]  KtParamMax=[]  KbOutMin=[]  KbOutMax=[]  KtOutMin=[]  KtOutMax=[]  IntegratorOutMin=[]  IntegratorOutMax=[]  FilterOutMin=[]  FilterOutMax=[]  SumI1OutMin=[]  SumI1OutMax=[]  SumI2OutMin=[]  SumI2OutMax=[]  SumI3OutMin=[]  SumI3OutMax=[]  SumI4OutMin=[]  SumI4OutMax=[]  SumDOutMin=[]  SumDOutMax=[]  DifferentiatorOutMin=[]  DifferentiatorOutMax=[]  FilterDiffOutCoefMin=[]  FilterDiffOutCoefMax=[]  ReciprocalOutMin=[]  ReciprocalOutMax=[]  SumDenOutMin=[]  SumDenOutMax=[]  SumNumOutMin=[]  SumNumOutMax=[]  DivideOutMin=[]  DivideOutMax=[]  IntegratorContinuousStateAttributes=''  IntegratorStateMustResolveToSignalObject=off  IntegratorRTWStateStorageClass=Auto  FilterContinuousStateAttributes=''  FilterStateMustResolveToSignalObject=off  FilterRTWStateStorageClass=Auto  ParallelPVariant=InternalParameters  IdealPVariant=Disabled  IVariant=InternalParameters  DVariant=Disabled  IntegratorVariant=Discrete  SatVariant=Disabled  AWVariant=Passthrough  PCopyVariant=Disabled  TRVariant=Disabled  FdbkBlocksVariant=Forward  IdealPFdbkVariant=Disabled  SatFdbkVariant=Disabled  DerivativeFilterVariant=Disabled  NVariant=Disabled  NCopyVariant=Disabled_SignalSpec  FilterICVariant=Disabled  IntegratorICVariant=InternalICs  ExternalResetVariant=Disabled  TRSumVariant=Passthrough  SumFdbkVariant=Disabled  SumVariant=Sum_PI
  filter : Subsystem
  filter1 : Subsystem
  filter2 : Subsystem
  filter3 : Subsystem
  filter4 : Subsystem
  filter5 : Subsystem
  servo_Tref : Outport  Unit=N*m
  wires:
  [servo1_qdref] -> filter/1(reference)
  [servo1_Tref] -> Mux/1
  Demux1/1 -> Gain4/1
  Gain2/1 -> [servo1_qdref]
  Gain6/1 -> [servo3_qdref]
  Gain12/1 -> [servo5_qdref]
  filter4/1(control) -> PID Controller3/1
  Gain15/1 -> [servo6_qdref]
  Demux/5 -> Gain12/1
  Gain5/1 -> [joint2_qd]
  Demux1/4 -> Gain10/1
  Gain13/1 -> [joint5_qd]
  Gain16/1 -> [joint6_qd]
  PID Controller5/1 -> [servo6_Tref]
  [servo6_qdref] -> filter5/1(reference)
  Gain10/1 -> [joint4_qd]
  [servo2_qdref] -> filter1/1(reference)
  Demux1/6 -> Gain16/1
  [servo2_Tref] -> Mux/2
  Gain3/1 -> [servo2_qdref]
  Gain9/1 -> [servo4_qdref]
  Gain7/1 -> [joint3_qd]
  [joint3_qd] -> filter2/2(output)
  Gain4/1 -> [joint1_qd]
  filter1/1(control) -> PID Controller2/1
  [servo4_Tref] -> Mux/4
  [joint5_qd] -> filter4/2(output)
  [servo3_Tref] -> Mux/3
  Demux1/5 -> Gain13/1
  Demux1/2 -> Gain5/1
  Demux/4 -> Gain9/1
  Mux/1 -> servo_Tref/1  "torqueReference"
  joint_qd/1 -> Demux1/1
  [servo4_qdref] -> filter3/1(reference)
  Demux1/3 -> Gain7/1
  [servo3_qdref] -> filter2/1(reference)
  [servo5_Tref] -> Mux/5
  [servo6_Tref] -> Mux/6
  servon_qdref/1 -> Demux/1
  Demux/1 -> Gain2/1
  Demux/6 -> Gain15/1
  [joint2_qd] -> filter1/2(output)
  [joint6_qd] -> filter5/2(output)
  Demux/2 -> Gain3/1
  Demux/3 -> Gain6/1
  PID Controller3/1 -> [servo5_Tref]
  PID Controller2/1 -> [servo2_Tref]
  filter5/1(control) -> PID Controller5/1
  PID Controller4/1 -> [servo3_Tref]
  filter2/1(control) -> PID Controller4/1
  PID Controller1/1 -> [servo4_Tref]
  filter3/1(control) -> PID Controller1/1
  PID Controller/1 -> [servo1_Tref]
  filter/1(control) -> PID Controller/1
  [joint4_qd] -> filter3/2(output)
  [joint1_qd] -> filter/2(output)
  [servo5_qdref] -> filter4/1(reference)

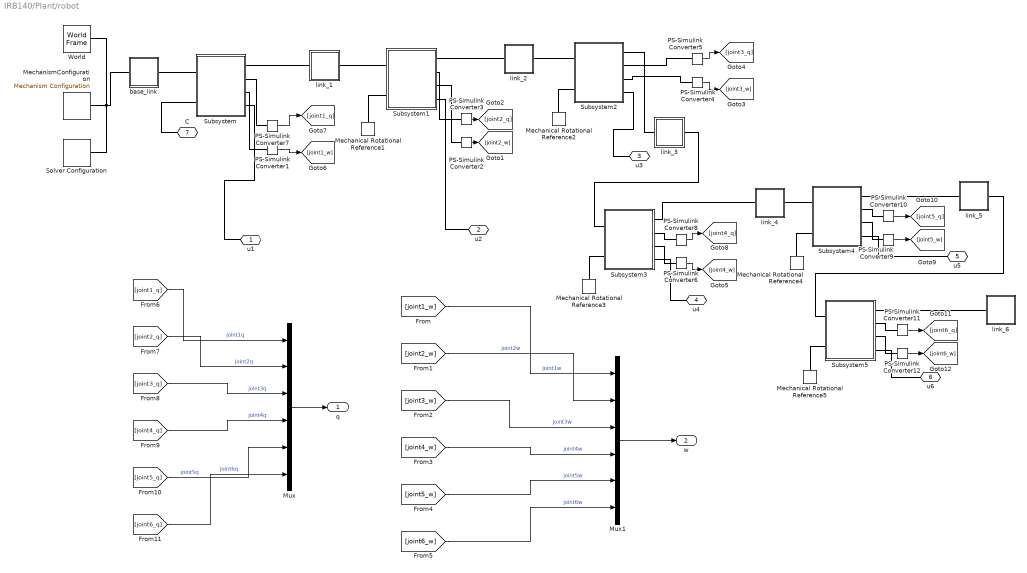
== system IRB140/Plant/robot ==
  Mechanical Rotational Reference{1..5} (5 alike) : fl_lib/Mechanical/Rotational Elements/Mechanical Rotational Reference
  MechanismConfiguration : sm_lib/Utilities/Mechanism Configuration  UniformGravity=Constant  GravityVector=[0 0 0]  GravityUnits=m/s^2  LinearizationDelta=0.001
  Mux : Mux  Inputs=6
  Mux1 : Mux  Inputs=6
  PS-Simulink Converter{1..2,4,6,9,12} (6 alike) : nesl_utility/PS-Simulink Converter  PhysicalDomain=network_engine_domain  SubClassName=ps_output  LeftPortType=input  RightPortType=output  PseudoPeriodic=off  Frequencies=[]  Unit=deg/s  AffineConversion=off
  PS-Simulink Converter{3,5,7..8,10..11} (6 alike) : nesl_utility/PS-Simulink Converter  PhysicalDomain=network_engine_domain  SubClassName=ps_output  LeftPortType=input  RightPortType=output  PseudoPeriodic=off  Frequencies=[]  Unit=deg  AffineConversion=off
  Solver Configuration : nesl_utility/Solver Configuration  PhysicalDomain=network_engine_domain  SubClassName=solver  LeftPortType=input  RightPortType=generic  Tones=[]  Harmonics=[]  SimulateNoise=off  Profile=off  UseLocalSampling=off  EnableSwitchedLinearOptims=on  FrequencyDomain=off  UseCCode=off  RelTol=0.001  AbsTol=1e-06  MinStep=1e-09  ToWorkspace=off  RevertToSquareIcSolve=off  NumHomotopyIterations=100  PhasorMode=off  PhasorModeNumHarmonics=1  DoDC=off  ResidualTolerance=1e-09  UseLocalSolver=off  LocalSolverChoice=NE_BACKWARD_EULER_ADVANCER  LocalSolverSampleTime=0.001  DoFixedCost=off  MaxNonlinIter=3  MaxModeIter=2  LinearAlgebra=auto  EquationFormulation=NE_TIME_EF  DelaysMemoryBudget=1024  AutomaticFiltering=on  FilteringTimeConstant=0.001  PartitionStorageMethod=AS_NEEDED  PartitionMemoryBudget=1024  PartitionMethod=ROBUST
  Subsystem : Subsystem
  Subsystem1 : Subsystem
  Subsystem2 : Subsystem
  Subsystem3 : Subsystem
  Subsystem4 : Subsystem
  Subsystem5 : Subsystem
  World : sm_lib/Frames and Transforms/World Frame
  base_link : Subsystem
  link_1 : Subsystem
  link_2 : Subsystem
  link_3 : Subsystem
  link_4 : Subsystem
  link_5 : Subsystem
  link_6 : Subsystem
  u1 : PMIOPort  Side=Left
  u2 : PMIOPort  Port=2  Side=Left
  u3 : PMIOPort  Port=3  Side=Left
  u4 : PMIOPort  Port=4  Side=Left
  u5 : PMIOPort  Port=5  Side=Left
  u6 : PMIOPort  Port=6  Side=Left
  C : PMIOPort  Port=7  Side=Left
  q : Outport  Unit=deg
  w : Outport  Port=2  Unit=deg/s
  wires:
  [joint2_w] -> Mux1/2  "joint2w"
  PS-Simulink Converter1/1 -> [joint1_w]
  [joint4_q] -> Mux/4  "joint4q"
  [joint6_w] -> Mux1/6  "joint6w"
  PS-Simulink Converter8/1 -> [joint4_q]
  PS-Simulink Converter4/1 -> [joint3_w]
  [joint1_w] -> Mux1/1  "joint1w"
  [joint2_q] -> Mux/2  "joint2q"
  PS-Simulink Converter12/1 -> [joint6_w]
  PS-Simulink Converter11/1 -> [joint6_q]
  [joint5_q] -> Mux/5  "joint5q"
  [joint6_q] -> Mux/6  "joint6q"
  Mux1/1 -> w/1
  PS-Simulink Converter3/1 -> [joint2_q]
  [joint1_q] -> Mux/1  "joint1q"
  [joint3_q] -> Mux/3  "joint3q"
  PS-Simulink Converter9/1 -> [joint5_w]
  PS-Simulink Converter7/1 -> [joint1_q]
  PS-Simulink Converter10/1 -> [joint5_q]
  [joint5_w] -> Mux1/5  "joint5w"
  PS-Simulink Converter5/1 -> [joint3_q]
  Mux/1 -> q/1
  PS-Simulink Converter6/1 -> [joint4_w]
  PS-Simulink Converter2/1 -> [joint2_w]
  [joint4_w] -> Mux1/4  "joint4w"
  [joint3_w] -> Mux1/3  "joint3w"
  connections:
  Subsystem4/LConn1 -- link_4/RConn1
  World/RConn1 -- MechanismConfiguration/RConn1 -- Solver Configuration/RConn1 -- base_link/LConn1
  Mechanical Rotational Reference3/LConn1 -- Subsystem3/LConn2
  Subsystem4/RConn1 -- link_5/LConn1
  PS-Simulink Converter8/LConn1 -- Subsystem3/RConn2
  u4/RConn1 -- Subsystem3/RConn4
  PS-Simulink Converter12/LConn1 -- Subsystem5/RConn3
  PS-Simulink Converter11/LConn1 -- Subsystem5/RConn2
  Mechanical Rotational Reference4/LConn1 -- Subsystem4/LConn2
  PS-Simulink Converter1/LConn1 -- Subsystem/RConn3
  Mechanical Rotational Reference5/LConn1 -- Subsystem5/LConn2
  u3/RConn1 -- Subsystem2/RConn4
  Subsystem2/LConn1 -- link_2/RConn1
  u2/RConn1 -- Subsystem1/RConn4
  C/RConn1 -- Subsystem/LConn2
  Subsystem2/RConn1 -- link_3/LConn1
  PS-Simulink Converter10/LConn1 -- Subsystem4/RConn2
  PS-Simulink Converter6/LConn1 -- Subsystem3/RConn3
  u5/RConn1 -- Subsystem4/RConn4
  PS-Simulink Converter3/LConn1 -- Subsystem1/RConn2
  PS-Simulink Converter7/LConn1 -- Subsystem/RConn2
  PS-Simulink Converter5/LConn1 -- Subsystem2/RConn2
  link_2/LConn1 -- Subsystem1/RConn1
  Subsystem3/RConn1 -- link_4/LConn1
  link_1/RConn1 -- Subsystem1/LConn1
  base_link/RConn1 -- Subsystem/LConn1
  PS-Simulink Converter2/LConn1 -- Subsystem1/RConn3
  Subsystem3/LConn1 -- link_3/RConn1
  Subsystem/RConn1 -- link_1/LConn1
  Subsystem5/LConn1 -- link_5/RConn1
  PS-Simulink Converter9/LConn1 -- Subsystem4/RConn3
  u1/RConn1 -- Subsystem/RConn4
  PS-Simulink Converter4/LConn1 -- Subsystem2/RConn3
  u6/RConn1 -- Subsystem5/RConn4
  Subsystem5/RConn1 -- link_6/LConn1
  Mechanical Rotational Reference2/LConn1 -- Subsystem2/LConn2
  Subsystem1/LConn2 -- Mechanical Rotational Reference1/LConn1

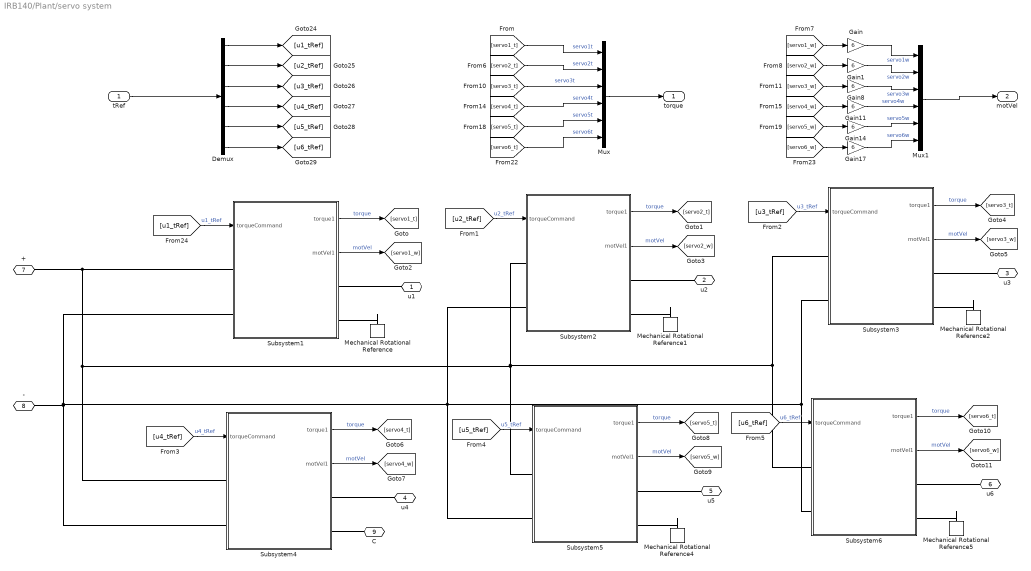
== system IRB140/Plant/servo system ==
  tRef : Inport  Unit=N*m
  Demux : Demux  Outputs=6
  Gain{,1,8,11,14,17} (6 alike) : Gain  Gain=6
  Mechanical Rotational Reference{,1..2,4..5} (5 alike) : fl_lib/Mechanical/Rotational Elements/Mechanical Rotational Reference
  Mux : Mux  Inputs=6
  Mux1 : Mux  Inputs=6
  Subsystem1 : Subsystem
  Subsystem2 : Subsystem
  Subsystem3 : Subsystem
  Subsystem4 : Subsystem
  Subsystem5 : Subsystem
  Subsystem6 : Subsystem
  u1 : PMIOPort  Side=Right
  u2 : PMIOPort  Port=2  Side=Right
  u3 : PMIOPort  Port=3  Side=Right
  u4 : PMIOPort  Port=4  Side=Right
  u5 : PMIOPort  Port=5  Side=Right
  u6 : PMIOPort  Port=6  Side=Right
  + : PMIOPort  Port=7  Side=Left
  - : PMIOPort  Port=8  Side=Left
  C : PMIOPort  Port=9  Side=Right
  torque : Outport  Unit=N*m
  motVel : Outport  Port=2  Unit=deg/s
  wires:
  [u6_tRef] -> Subsystem6/1(torqueCommand)  "u6_tRef"
  [u3_tRef] -> Subsystem3/1(torqueCommand)  "u3_tRef"
  Gain1/1 -> Mux1/2  "servo2w"
  [servo2_w] -> Gain1/1
  [servo6_w] -> Gain17/1
  [u2_tRef] -> Subsystem2/1(torqueCommand)  "u2_tRef"
  [servo1_w] -> Gain/1
  [servo4_w] -> Gain11/1
  Subsystem5/1(torque1) -> [servo5_t]  "torque"
  Subsystem4/2(motVel1) -> [servo4_w]  "motVel"
  Gain11/1 -> Mux1/4  "servo4w"
  Subsystem3/1(torque1) -> [servo3_t]  "torque"
  [servo3_w] -> Gain8/1
  [servo5_w] -> Gain14/1
  Subsystem6/2(motVel1) -> [servo6_w]  "motVel"
  Subsystem6/1(torque1) -> [servo6_t]  "torque"
  Subsystem3/2(motVel1) -> [servo3_w]  "motVel"
  Subsystem5/2(motVel1) -> [servo5_w]  "motVel"
  Gain/1 -> Mux1/1  "servo1w"
  Subsystem4/1(torque1) -> [servo4_t]  "torque"
  [u1_tRef] -> Subsystem1/1(torqueCommand)  "u1_tRef"
  Gain17/1 -> Mux1/6  "servo6w"
  Mux1/1 -> motVel/1
  Subsystem2/2(motVel1) -> [servo2_w]  "motVel"
  Subsystem2/1(torque1) -> [servo2_t]  "torque"
  Gain8/1 -> Mux1/3  "servo3w"
  [u5_tRef] -> Subsystem5/1(torqueCommand)  "u5_tRef"
  Subsystem1/1(torque1) -> [servo1_t]  "torque"
  [u4_tRef] -> Subsystem4/1(torqueCommand)  "u4_tRef"
  Subsystem1/2(motVel1) -> [servo1_w]  "motVel"
  Gain14/1 -> Mux1/5  "servo5w"
  Demux/1 -> [u1_tRef]
  Demux/2 -> [u2_tRef]
  Demux/3 -> [u3_tRef]
  Demux/4 -> [u4_tRef]
  Demux/5 -> [u5_tRef]
  Demux/6 -> [u6_tRef]
  tRef/1 -> Demux/1
  Mux/1 -> torque/1
  [servo1_t] -> Mux/1  "servo1t"
  [servo2_t] -> Mux/2  "servo2t"
  [servo3_t] -> Mux/3  "servo3t"
  [servo4_t] -> Mux/4  "servo4t"
  [servo5_t] -> Mux/5  "servo5t"
  [servo6_t] -> Mux/6  "servo6t"
  connections:
  Mechanical Rotational Reference5/LConn1 -- Subsystem6/RConn2
  u4/RConn1 -- Subsystem4/RConn1
  u3/RConn1 -- Subsystem3/RConn1
  u6/RConn1 -- Subsystem6/RConn1
  Subsystem1/LConn2 -- -/RConn1 -- Subsystem4/LConn2 -- Subsystem6/LConn2 -- Subsystem3/LConn2 -- Subsystem5/LConn2 -- Subsystem2/LConn2
  Mechanical Rotational Reference2/LConn1 -- Subsystem3/RConn2
  u2/RConn1 -- Subsystem2/RConn1
  Subsystem1/LConn1 -- +/RConn1 -- Subsystem5/LConn1 -- Subsystem3/LConn1 -- Subsystem6/LConn1 -- Subsystem2/LConn1 -- Subsystem4/LConn1
  u1/RConn1 -- Subsystem1/RConn1
  Mechanical Rotational Reference/LConn1 -- Subsystem1/RConn2
  Mechanical Rotational Reference1/LConn1 -- Subsystem2/RConn2
  Mechanical Rotational Reference4/LConn1 -- Subsystem5/RConn2
  u5/RConn1 -- Subsystem5/RConn1
  Subsystem4/RConn2 -- C/RConn1

== system IRB140/r/Subsystem ==
  Sine Wave : Sin  Amplitude=50
  Sine Wave1 : Sin  Amplitude=40
  Sine Wave2 : Sin  Amplitude=20
  Sine Wave3 : Sin  Amplitude=20
  Sine Wave4 : Sin  Amplitude=150
  Sine Wave5 : Sin  Amplitude=100
  Out1 : Outport
  Out2 : Outport  Port=2
  Out3 : Outport  Port=3
  Out4 : Outport  Port=4
  Out5 : Outport  Port=5
  Out6 : Outport  Port=6
  wires:
  Sine Wave3/1 -> Out4/1
  Sine Wave1/1 -> Out2/1
  Sine Wave4/1 -> Out5/1
  Sine Wave5/1 -> Out6/1
  Sine Wave2/1 -> Out3/1
  Sine Wave/1 -> Out1/1
